simulink library "GF1_Blocks"  (R2021b)
settings: Solver=VariableStepAuto  StartTime=0.0  StopTime=10.0  RelTol=1e-3
settings Model: Creator=Edwar  LastModifiedBy=Edwar

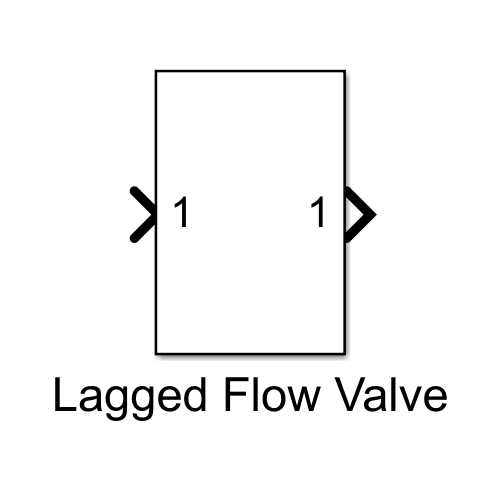
[thumbnail: Simulink's stored preview of the top-level diagram]
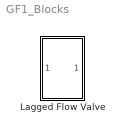
== system GF1_Blocks ==
  Lagged Flow Valve : Subsystem

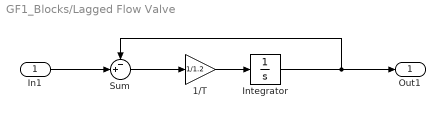
== system GF1_Blocks/Lagged Flow Valve ==
  In1 : Inport
  1/T : Gain  Gain=1/1.2
  Integrator : Integrator
  Sum : Sum  Inputs=-+|
  Out1 : Outport
  wires:
  Integrator/1 -> Out1/1, Sum/1
  Sum/1 -> 1/T/1
  1/T/1 -> Integrator/1
  In1/1 -> Sum/2
